simulink model "z_gen1"  (Simulink 3.00)
settings: Solver=ode45  StartTime=0.0  StopTime=sum(inter)  RelTol=1e-3
values from neighbouring files (symbols this model uses):
  i = i+1    (= 2)    [clink.m]
undefined symbols (not defined in the file or in its folder): cuminter, inter

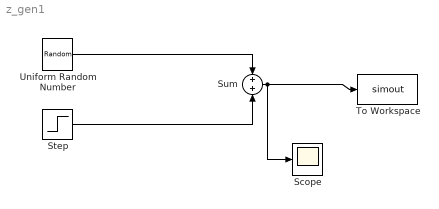
== system z_gen1 ==
  Scope : Scope
      settings: TimeRange=auto  YMin=-5  YMax=5  SaveToWorkspace=off  SaveName=ScopeData
  Step : Step  Time=cuminter(i)  Before=0  After=rand*3  SampleTime=0
  Sum : Sum  Inputs=+|+  SaturateOnIntegerOverflow=on
  To Workspace : ToWorkspace  VariableName=simout  SampleTime=1  SaveFormat=Matrix
  Uniform Random Number : UniformRandomNumber  Minimum=0.1  Maximum=1  Seed=rand  SampleTime=min(inter)/(rand*10)
  wires:
  Uniform Random Number/1 -> Sum/1
  Step/1 -> Sum/2
  Sum/1 -> To Workspace/1, Scope/1
